simulink model "xpcrs232V2"  (Simulink 5.0)
settings: Solver=ode5  StartTime=0.0  StopTime=300  RelTol=1e-3
PreLoadFcn:
  | RS232Async_Messages
libraries: xpclib x5
settings Model: LastModifiedBy=vsriniva  ExtModeMexFile=ext_xpc  ExtModeArmWhenConnect=off  SaveState=on  LimitDataPoints=off  OptimizeBlockIOStorage=off  RTWSystemTargetFile=xpctarget.tlc  RTWTemplateMakefile=xpc_default_tmf  RTWOptions="-aEnforceIntegerDowncast=0 -aExtMode=1 -aFoldNonRolledExpr=0 -aForceParamTrailComments=0 -aGenerateComments=1 -aGenerateReport=0 -aIncDataTypeInIds=0 -aIncHierarchyInIds=0 -aInlineInvariantSignals=0 -aInlineParameters=0 -aInlinedPrmAccess=\"Literals\" -aLocalBlockOutputs=0 -aMaxRTWIdLen=31 -aPrefixModelToSubsysFcnNames=1 -aRL32IRQSourceModifier=\"Timer\" -aRL32LogBufSizeModifier=100000 -aRL32LogTETModifier=1 -aRL32ModeModifier=\"Real-Time\" -aRL32ObjectName=\"tg\" -aRTWVerbose=1 -aRollThreshold=5 -aShowEliminatedStatements=0 -axPCIOIRQSlot=-1 -axPCIRQSourceBoard=\"None/Other\" -axpcDblBuff=0 -axpcObjCom=0"

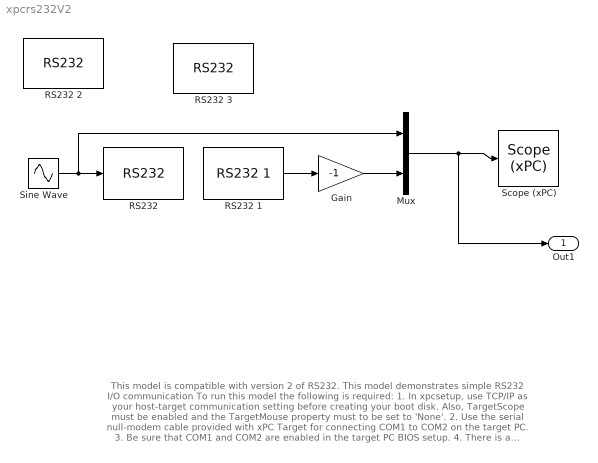
== system xpcrs232V2 ==
  note: This  model is compatible with version 2 of RS232.
      |
      | This model demonstrates simple RS232 I/O communication
      |
      | To run this model the following is required:
      |
      | 1. In xpcsetup, use TCP/IP as your host-target communication setting before creating your boot disk.
      | Also, TargetScope must be enabled and the TargetMouse property must to be set to 'None'.
      |
      | 2. Use the serial null-modem cable provided with xPC Target for connecting COM1 to
      | COM2 on the target PC.
      |
      | 3. Be sure that COM1 and COM2 are enabled in the target PC BIOS setup.
      |
      | 4. There is a preloaded function associated with the send/receive blocks. Look for RS232Async_Messages.m
      |
      | 5.If you do not manually load the message structures before opening your Simulink model, or have the message
      |    structures automatically loaded with the model, the port connections to the RS-232 blocks break.
  Gain : Gain  Gain=-1  SaturateOnIntegerOverflow=on
  Mux : Mux  Inputs=2
  "RS232 " : xpclib/RS232/Asynchronous Mode/RS232   port=COM1  blockvar=RS232_Send  ts=0.1
  RS232 1 : xpclib/RS232/Asynchronous Mode/RS232 1  port=COM2  blockvar=RS232_Receive  ts=0.1
  RS232 2 : xpclib/RS232/RS232   port=COM1  baud=115200  dbits=8  sbits=1  parity=None  prot=None  sbuf=1024  rbuf=1024  initstruct=[]  termstruct=[]
  RS232 3 : xpclib/RS232/RS232   port=COM2  baud=115200  dbits=8  sbits=1  parity=None  prot=None  sbuf=1024  rbuf=1024  initstruct=[]  termstruct=[]
  "Scope (xPC) " : xpclib/Misc./Scope (xPC)   scopeno=1  scopetype=Target  viewmode=Graphical rolling  grid=on  ylimits=[0,0]  autostart=on  nosamples=250  noprepostsamples=0  interleave=1  triggermode=FreeRun  triggersignal=1  triggerlevel=0.0  triggerslope=either  triggerscope=1  triggersample=0
  Sine Wave : Sin  Frequency=5  SampleTime=0
  Out1 : Outport
  wires:
  RS232 1/1 -> Gain/1
  Gain/1 -> Mux/2
  Mux/1 -> "Scope (xPC) "/1, Out1/1
  Sine Wave/1 -> Mux/1, "RS232 "/1
